simulink model "task1"  (R2025b)
settings: Solver=VariableStepAuto  StartTime=0.0  StopTime=24  RelTol=1e-3
values from neighbouring files (symbols this model uses):
  Sb_0 = 0.55    [init.m]
  Ta_0 = 10.0    (= 10)    [init.m]
  Tp_0 = 11.5    [init.m]
settings Model: Creator=davide  LastModifiedBy=davide

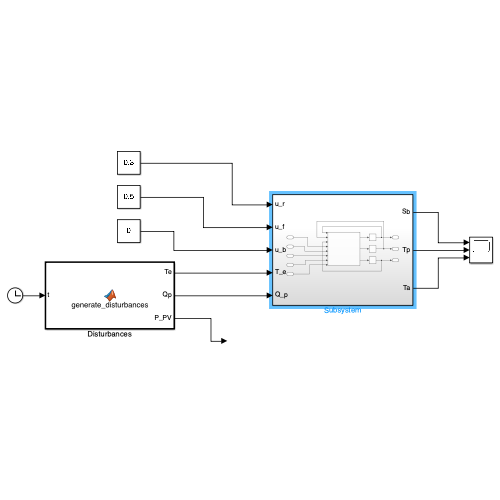
[thumbnail: Simulink's stored preview of the top-level diagram]
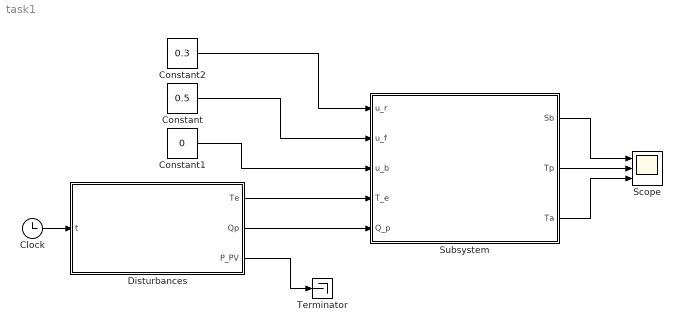
== system task1 ==
  Clock : Clock
  Constant : Constant  Value=0.5
  Constant1 : Constant  Value=0
  Constant2 : Constant  Value=0.3
  Disturbances : MATLAB Function  TreatAsAtomicUnit=on
  Scope : Scope  NumInputPorts=3
      settings: ActiveDisplayYMinimum=-1.1983578300290532  ActiveDisplayYMaximum=16.285220470261482
  Subsystem : Subsystem
  Terminator : Terminator
  wires:
  Clock/1 -> Disturbances/1(t)
  Disturbances/1(Te) -> Subsystem/4(T_e)
  Disturbances/2(Qp) -> Subsystem/5(Q_p)
  Constant2/1 -> Subsystem/1(u_r)
  Constant/1 -> Subsystem/2(u_f)
  Constant1/1 -> Subsystem/3(u_b)
  Disturbances/3(P_PV) -> Terminator/1
  Subsystem/3(Ta) -> Scope/3
  Subsystem/2(Tp) -> Scope/2
  Subsystem/1(Sb) -> Scope/1

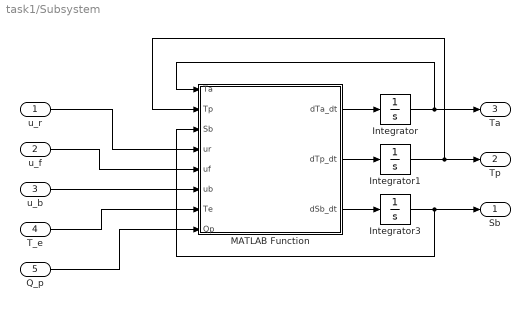
== system task1/Subsystem ==
  u_r : Inport
  u_f : Inport  Port=2
  u_b : Inport  Port=3
  T_e : Inport  Port=4
  Q_p : Inport  Port=5
  Integrator : Integrator  InitialCondition=Ta_0
  Integrator1 : Integrator  InitialCondition=Tp_0
  Integrator3 : Integrator  InitialCondition=Sb_0
  MATLAB Function : MATLAB Function  TreatAsAtomicUnit=on
  Sb : Outport
  Tp : Outport  Port=2
  Ta : Outport  Port=3
  wires:
  MATLAB Function/1(dTa_dt) -> Integrator/1
  MATLAB Function/2(dTp_dt) -> Integrator1/1
  MATLAB Function/3(dSb_dt) -> Integrator3/1
  Integrator3/1 -> Sb/1, MATLAB Function/3(Sb)
  Integrator/1 -> Ta/1, MATLAB Function/1(Ta)
  Integrator1/1 -> MATLAB Function/2(Tp), Tp/1
  u_r/1 -> MATLAB Function/4(ur)
  u_f/1 -> MATLAB Function/5(uf)
  u_b/1 -> MATLAB Function/6(ub)
  T_e/1 -> MATLAB Function/7(Te)
  Q_p/1 -> MATLAB Function/8(Qp)

== matlab function task1/Disturbances ==
  data: t input; Te output; Qp output; P_PV output
function [Te, Qp, P_PV] = generate_disturbances(t)
    Rmax = 850; Pmax = 9.0;
    
    Te = 24 + 8 * sin(pi/12 * (t - 8));
    
    if t >= 6 && t <= 18
        Rs = Rmax * sin(pi * (t - 6) / 12);
    else
        Rs = 0;
    end
    P_PV = Pmax * (Rs / Rmax);
    
    % Thermal Charge   
    if t < 4
        Qp = 1200;
    elseif t < 10
        Qp = 600;
    else
        Qp = 250;
    end
end

== matlab function task1/Subsystem/MATLAB Function ==
  data: Ta input; dTa_dt output; Tp input; Sb input; ur input; uf input; ub input; Te input; Qp input; dTp_dt output; dSb_dt output
function [dTa_dt, dTp_dt, dSb_dt] = plant_equations(Ta, Tp, Sb, ur, uf, ub, Te, Qp)
    Ca = 1.5e5; Cp = 8.0e5; ke = 3.8*70; kr = 1.6e4; kf = 450; alpha_f = 1.0;
    Eb = 18; eta_b = 0.94; sec2hour = 3600;

    % Saturations
    ur = max(0, min(1, ur));
    uf = max(0, min(1, uf));
    ub = max(-4, min(4, ub));
    
    if (Sb <= 0.15 && ub < 0) || (Sb >= 0.95 && ub > 0)
        ub = 0; 
    end

    % sec2hour
    dTa_dt = (sec2hour / Ca) * (ke * (Te - Ta) - kr * ur - kf * (1 + alpha_f * uf) * (Ta - Tp) + Qp);
    dTp_dt = (sec2hour / Cp) * (kf * (1 + alpha_f * uf) * (Ta - Tp));
    dSb_dt = (1 / Eb) * ( -(1 / eta_b) * max(-ub, 0) - eta_b * max(ub, 0) );
end
